simulink model "GFLIB_Hyst_BAM_FLT"  (Simulink 7.3)
settings: Solver=ode45  StartTime=0.0  StopTime=10.0  RelTol=1e-3
undefined symbols (not defined in the file): fltHystOff, fltHystOn, fltOutValOff, fltOutValOn
settings Model: Creator=B17364  LastModifiedBy=B17364

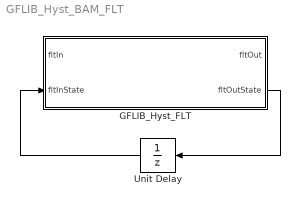
== system GFLIB_Hyst_BAM_FLT ==
  GFLIB_Hyst_FLT : Subsystem  mask(GFLIB_Hyst_FLT){fltHystOn=fltHystOn, fltHystOff=fltHystOff, fltOutValOn=fltOutValOn, fltOutValOff=fltOutValOff}
      mask help: Bit accurate model of hysteresis function. All parameters as well as input and output are in a full float range.
      mask init:
      | pos = get_param(gcb, 'Position');width = pos(3) - pos(1); height = pos(4) - pos(2);tX=width/2;tY=height*0.9;
      mask Display: color('black');port_label('input',1,'fltIn');port_label('input',2,'fltInState');port_label('output',1,'fltOut');port_label('output',2,'fltOutState');color('black');disp('GFLIB_Hyst_FLT');color('blue');text(tX,tY, 'BAM', 'horizontalAlignment', 'center');
  Unit Delay : UnitDelay  SampleTime=-1
  wires:
  GFLIB_Hyst_FLT/2(fltOutState) -> Unit Delay/1
  Unit Delay/1 -> GFLIB_Hyst_FLT/2(fltInState)

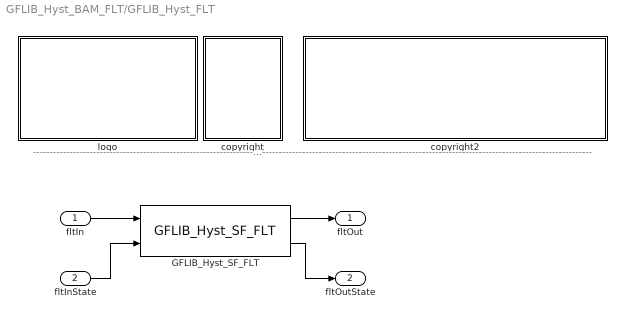
== system GFLIB_Hyst_BAM_FLT/GFLIB_Hyst_FLT ==
  note: ---------------------------------------------------------------------------------------------------------------------------------------------------------------------------------------------------
  fltIn : Inport  OutDataType=fixdt(1, 16)  OutScaling=2^0
  fltInState : Inport  Port=2  OutDataType=fixdt(1, 16)  OutScaling=2^0
  GFLIB_Hyst_SF_FLT : S-Function  FunctionName=GFLIB_Hyst_SF_FLT  Parameters=fltHystOn,fltHystOff,fltOutValOn,fltOutValOff  EnableBusSupport=off
  copyright : Subsystem
      mask Display: text(10,90,'FILE:');text(10,75,'DESRIPTION:')text(10,60,'COPYRIGHT:')text(10,45,'VERSION:')text(10,30,'DATE:')
  copyright2 : Subsystem
      mask Display: text(10,90,'GFLIB_Hyst_BAM_FLT.mdl');text(10,75,'Hysteresis function.');text(10,60,'Freescale')text(10,45,'0.1');text(10,30,'09-Apr-2014');
  logo : Subsystem
      mask Display: image(imread('logo.jpg'))
  fltOut : Outport  OutDataType=fixdt(1, 16)  OutScaling=2^0
  fltOutState : Outport  Port=2  OutDataType=fixdt(1, 16)  OutScaling=2^0
  wires:
  fltIn/1 -> GFLIB_Hyst_SF_FLT/1
  GFLIB_Hyst_SF_FLT/1 -> fltOut/1
  fltInState/1 -> GFLIB_Hyst_SF_FLT/2
  GFLIB_Hyst_SF_FLT/2 -> fltOutState/1

== system GFLIB_Hyst_BAM_FLT/GFLIB_Hyst_FLT/copyright ==

== system GFLIB_Hyst_BAM_FLT/GFLIB_Hyst_FLT/copyright2 ==

== system GFLIB_Hyst_BAM_FLT/GFLIB_Hyst_FLT/logo ==
